simulink model "simulacija2"  (R2015a)
settings: Solver=ode45  StartTime=0.0  StopTime=500  RelTol=1e-3
values from neighbouring files (symbols this model uses):
  C = C_r/m    (= 5.618808)    [parametri.m]
  K = 2*n*R_t/R    [parametri.m]
  n = 7    [parametri.m]
  R = R_r/m    [parametri.m]
  R_s1 = 1/(alfa_vaz*2*(a+b)*L/m)    (= 89.1265597148)    [parametri.m]
  R_s2 = 1/(alfa_vaz*a*b)    (= 1014.19878296)    [parametri.m]
  teta_k = 70    [parametri.m]
  teta_vaz = 30    [parametri.m]
settings Model: Creator=zracenje  LastModifiedBy=Danijel
settings DebuggingCC: UnderspecifiedInitializationDetection=Classic  MergeDetectMultiDrivingBlocksExec=none  SolverPrmCheckMsg=warning

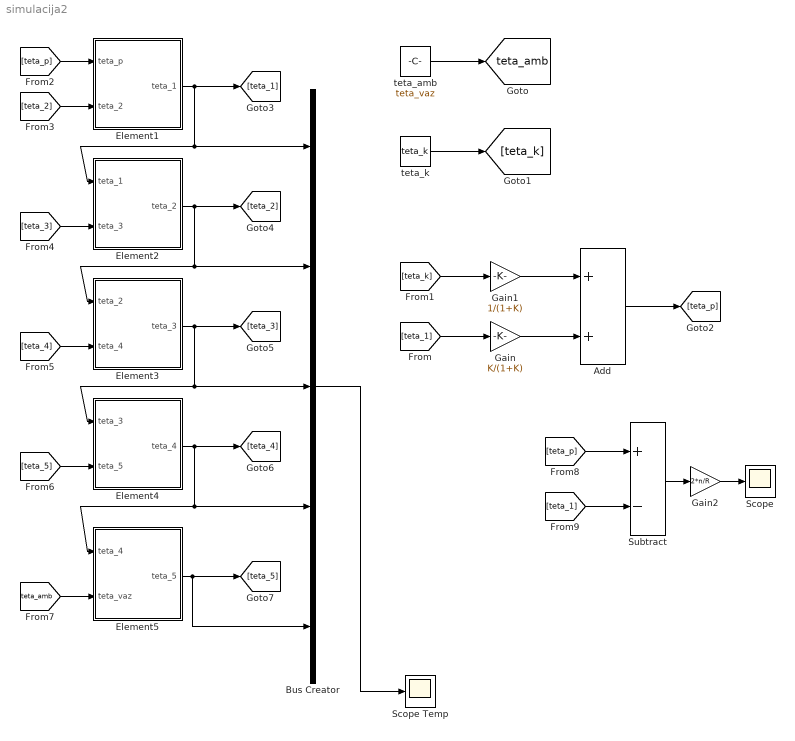
== system simulacija2 ==
  Add : Sum
  Bus Creator : BusCreator  Inputs=5
  Element1 : Subsystem
  Element2 : Subsystem
  Element3 : Subsystem
  Element4 : Subsystem
  Element5 : Subsystem
  Gain : Gain  Gain=K/(1+K)
  Gain1 : Gain  Gain=1/(1+K)
  Gain2 : Gain  Gain=2*n/R
  Scope : Scope
  Scope Temp : Scope
      settings: TimeRange=200  YMin=58.28979143798024  YMax=74.28979143798024
  Subtract : Sum  Inputs=+-
  teta_amb : Constant  Value=teta_vaz
  teta_k : Constant  Value=teta_k
  tag scope: teta_amb=global
  wires:
  teta_amb/1 -> [teta_amb]
  teta_k/1 -> [teta_k]
  Gain/1 -> Add/2
  [teta_1] -> Gain/1
  Gain1/1 -> Add/1
  [teta_k] -> Gain1/1
  Add/1 -> [teta_p]
  [teta_p] -> Element1/1(teta_p)
  Element1/1(teta_1) -> [teta_1], Bus Creator/1, Element2/1(teta_1)
  Element2/1(teta_2) -> [teta_2], Bus Creator/2, Element3/1(teta_2)
  Element3/1(teta_3) -> [teta_3], Bus Creator/3, Element4/1(teta_3)
  Element4/1(teta_4) -> [teta_4], Bus Creator/4, Element5/1(teta_4)
  [teta_amb] -> Element5/2(teta_vaz)
  [teta_5] -> Element4/2(teta_5)
  [teta_4] -> Element3/2(teta_4)
  [teta_3] -> Element2/2(teta_3)
  [teta_2] -> Element1/2(teta_2)
  [teta_1] -> Subtract/2
  [teta_p] -> Subtract/1
  Subtract/1 -> Gain2/1
  Gain2/1 -> Scope/1
  Element5/1(teta_5) -> Bus Creator/5, [teta_5]
  Bus Creator/1 -> Scope Temp/1

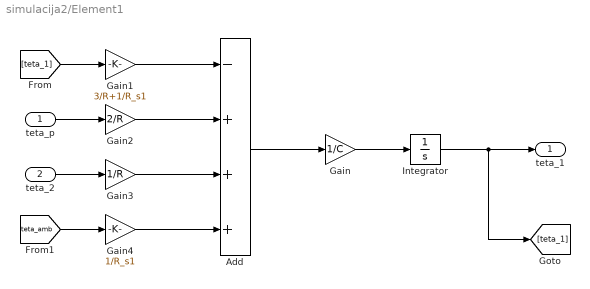
== system simulacija2/Element1 ==
  teta_p : Inport
  teta_2 : Inport  Port=2
  Add : Sum  Inputs=-+++
  Gain : Gain  Gain=1/C
  Gain1 : Gain  Gain=3/R+1/R_s1
  Gain2 : Gain  Gain=2/R
  Gain3 : Gain  Gain=1/R
  Gain4 : Gain  Gain=1/R_s1
  Integrator : Integrator  InitialCondition=teta_vaz
  teta_1 : Outport
  wires:
  teta_p/1 -> Gain2/1
  teta_2/1 -> Gain3/1
  Gain2/1 -> Add/2
  Gain4/1 -> Add/4
  Gain1/1 -> Add/1
  Integrator/1 -> [teta_1], teta_1/1
  Gain3/1 -> Add/3
  Add/1 -> Gain/1
  Gain/1 -> Integrator/1
  [teta_1] -> Gain1/1
  [teta_amb] -> Gain4/1

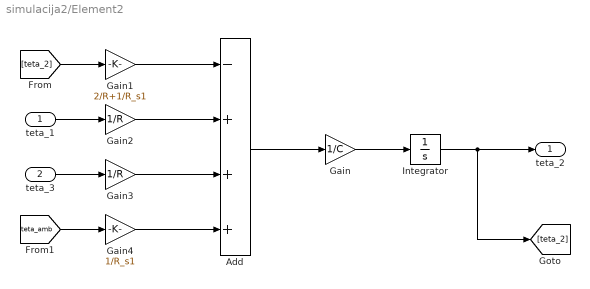
== system simulacija2/Element2 ==
  teta_1 : Inport
  teta_3 : Inport  Port=2
  Add : Sum  Inputs=-+++
  Gain : Gain  Gain=1/C
  Gain1 : Gain  Gain=2/R+1/R_s1
  Gain2 : Gain  Gain=1/R
  Gain3 : Gain  Gain=1/R
  Gain4 : Gain  Gain=1/R_s1
  Integrator : Integrator  InitialCondition=teta_vaz
  teta_2 : Outport
  wires:
  teta_1/1 -> Gain2/1
  teta_3/1 -> Gain3/1
  Gain2/1 -> Add/2
  Gain4/1 -> Add/4
  Gain1/1 -> Add/1
  Integrator/1 -> [teta_2], teta_2/1
  Gain3/1 -> Add/3
  Add/1 -> Gain/1
  Gain/1 -> Integrator/1
  [teta_2] -> Gain1/1
  [teta_amb] -> Gain4/1

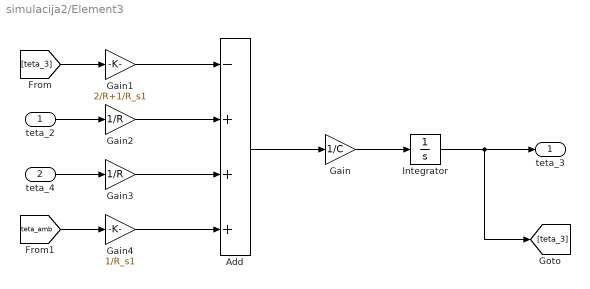
== system simulacija2/Element3 ==
  teta_2 : Inport
  teta_4 : Inport  Port=2
  Add : Sum  Inputs=-+++
  Gain : Gain  Gain=1/C
  Gain1 : Gain  Gain=2/R+1/R_s1
  Gain2 : Gain  Gain=1/R
  Gain3 : Gain  Gain=1/R
  Gain4 : Gain  Gain=1/R_s1
  Integrator : Integrator  InitialCondition=teta_vaz
  teta_3 : Outport
  wires:
  teta_2/1 -> Gain2/1
  teta_4/1 -> Gain3/1
  Gain2/1 -> Add/2
  Gain4/1 -> Add/4
  Gain1/1 -> Add/1
  Integrator/1 -> [teta_3], teta_3/1
  Gain3/1 -> Add/3
  Add/1 -> Gain/1
  Gain/1 -> Integrator/1
  [teta_3] -> Gain1/1
  [teta_amb] -> Gain4/1

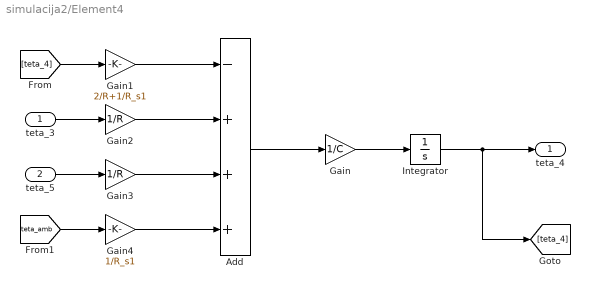
== system simulacija2/Element4 ==
  teta_3 : Inport
  teta_5 : Inport  Port=2
  Add : Sum  Inputs=-+++
  Gain : Gain  Gain=1/C
  Gain1 : Gain  Gain=2/R+1/R_s1
  Gain2 : Gain  Gain=1/R
  Gain3 : Gain  Gain=1/R
  Gain4 : Gain  Gain=1/R_s1
  Integrator : Integrator  InitialCondition=teta_vaz
  teta_4 : Outport
  wires:
  teta_3/1 -> Gain2/1
  teta_5/1 -> Gain3/1
  Gain2/1 -> Add/2
  Gain4/1 -> Add/4
  Gain1/1 -> Add/1
  Integrator/1 -> [teta_4], teta_4/1
  Gain3/1 -> Add/3
  Add/1 -> Gain/1
  Gain/1 -> Integrator/1
  [teta_4] -> Gain1/1
  [teta_amb] -> Gain4/1

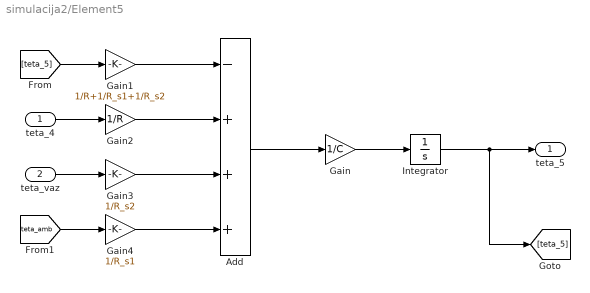
== system simulacija2/Element5 ==
  teta_4 : Inport
  teta_vaz : Inport  Port=2
  Add : Sum  Inputs=-+++
  Gain : Gain  Gain=1/C
  Gain1 : Gain  Gain=1/R+1/R_s1+1/R_s2
  Gain2 : Gain  Gain=1/R
  Gain3 : Gain  Gain=1/R_s2
  Gain4 : Gain  Gain=1/R_s1
  Integrator : Integrator  InitialCondition=teta_vaz
  teta_5 : Outport
  wires:
  teta_4/1 -> Gain2/1
  Gain2/1 -> Add/2
  Gain4/1 -> Add/4
  Gain1/1 -> Add/1
  Integrator/1 -> [teta_5], teta_5/1
  Gain3/1 -> Add/3
  Add/1 -> Gain/1
  Gain/1 -> Integrator/1
  [teta_5] -> Gain1/1
  [teta_amb] -> Gain4/1
  teta_vaz/1 -> Gain3/1
